simulink model "Comunicacao_Simulink_R2018b"  (R2018b)
settings: Solver=VariableStepAuto  StartTime=0.0  StopTime=10  RelTol=1e-3
libraries: dspsrcs4 x2, commsynccomp2 x1, simulink x1, dspmathops x1, commfilt2 x1, commutil2 x1
settings Model: Creator=rafae  LastModifiedBy=User

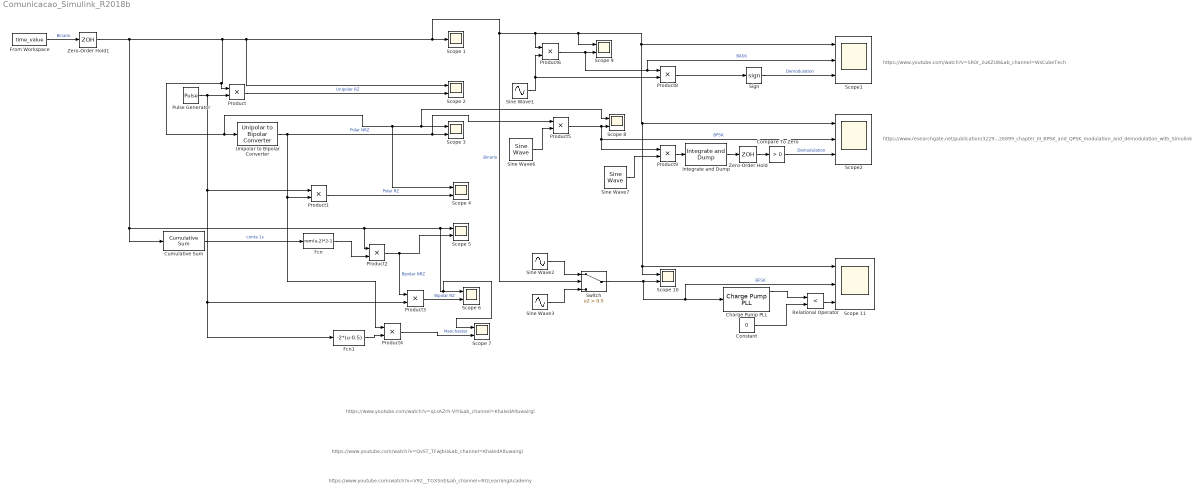
== system Comunicacao_Simulink_R2018b ==
  note: https://www.researchgate.net/publication/322926899_chapter_III_BPSK_and_QPSK_modulation_and_demodulation_with_Simulink
  note: https://www.youtube.com/watch?v=SR0r_2uKZU8&ab_channel=WsCubeTech
  note: https://www.youtube.com/watch?v=qLsAZrh-VIY&ab_channel=KhaledAltuwairgi
  note: https://www.youtube.com/watch?v=V92__TGXSnE&ab_channel=RGLearningAcademy
  note: https://www.youtube.com/watch?v=QvST_TFwJbU&ab_channel=KhaledAltuwairgi
  Charge Pump PLL : commsynccomp2/Charge Pump PLL  Fn=[2*pi*1]  Fd=[1 2*pi*1]  Kvco=4  Fc=10  Ph=0  Ac=1
      settings: SourceProductName=Communications Toolbox  SourceProductBaseCode=CM
  Compare To Zero : simulink/Logic and Bit Operations/Compare To Zero  relop=>  OutDataTypeStr=boolean
  Constant : Constant  Value=0
  Cumulative Sum : dspmathops/Cumulative Sum  dim=Channels (running sum)  InputProcessing=Columns as channels (frame based)  reset_popup=None  roundingMode=Floor  overflowMode=off  outputDataTypeStr=Inherit: Same as accumulator  outputMin=[]  outputMax=[]  outputLastDataTypeStr=Inherit: Same as accumulator
      settings: SourceProductName=DSP System Toolbox
  Fcn : Fcn  Expr=rem(u,2)*2-1
  Fcn1 : Fcn  Expr=-2*(u-0.5)
  From Workspace : FromWorkspace  VariableName=time_value  SampleTime=0
  Integrate and Dump : commfilt2/Integrate and Dump  obssamples=100  offsetsamples=0  nodump=on  roundingMode=Floor  overflowMode=off  outputDataTypeStr=Inherit: Same as accumulator  outputLastDataTypeStr=Inherit: Same as accumulator
      settings: SourceProductName=Communications Toolbox
  Product{,1..6,8..9} (9 alike) : Product
  Pulse Generator : DiscretePulseGenerator  PulseType=Time based  Period=1  PulseWidth=50
  Relational Operator : RelationalOperator  Operator=<  OutDataTypeStr=boolean  RndMeth=Simplest
  Scope 1 : Scope
  Scope {2..10} (9 alike) : Scope  NumInputPorts=2
  Scope 11 : Scope  NumInputPorts=3
  Scope1 : Scope  NumInputPorts=3
  Scope2 : Scope  NumInputPorts=3
  Sign : Signum
  Sine Wave1 : Sin  Frequency=2*pi*2  SampleTime=0
  Sine Wave2 : Sin  Frequency=2*pi*4  SampleTime=0
  Sine Wave3 : Sin  Frequency=2*pi*12  SampleTime=0
  Sine Wave6 : dspsrcs4/Sine Wave  Amplitude=1  Frequency=5  Phase=0  SampleMode=Discrete  OutComplex=Real  CompMethod=Trigonometric fcn  TableSize=Speed  SampleTime=1/1000  SamplesPerFrame=1  ResetState=Restart at time zero  OutputFrames=off  dataType=double  wordLen=16  udDataType=sfix(16)  fracBitsMode=Best precision  numFracBits=15  OutDataTypeStr=double  LastOutDataTypeStr=double
  Sine Wave7 : dspsrcs4/Sine Wave  Amplitude=1  Frequency=5  Phase=0  SampleMode=Discrete  OutComplex=Real  CompMethod=Trigonometric fcn  TableSize=Speed  SampleTime=1/1000  SamplesPerFrame=1  ResetState=Restart at time zero  OutputFrames=off  dataType=double  wordLen=16  udDataType=sfix(16)  fracBitsMode=Best precision  numFracBits=15  OutDataTypeStr=double  LastOutDataTypeStr=double
  Switch : Switch  Criteria=u2 > Threshold  Threshold=0.5
  Unipolar to Bipolar Converter : commutil2/Unipolar to Bipolar Converter  M=2  polarity=Positive  dataType=Inherit via internal rule
      settings: SourceProductName=Communications Toolbox
  Zero-Order Hold : ZeroOrderHold  SampleTime=-1
  Zero-Order Hold1 : ZeroOrderHold  SampleTime=-1
  wires:
  Zero-Order Hold1/1 -> Cumulative Sum/1, Product2/1, Scope 7/1, Scope 6/1, Scope 5/1, Scope 2/1, Switch/2, Scope2/1, Scope 10/1, Scope 11/1, Scope1/1, Scope 9/1, Product6/1, Scope 1/1, Scope 4/1, Scope 8/1, Scope 3/1, Unipolar to Bipolar Converter/1, Product/1  "Binario"
  Product/1 -> Scope 2/2  "Unipolar RZ"
  Unipolar to Bipolar Converter/1 -> Product4/1, Product1/2, Product5/1, Scope 3/2  "Polar NRZ"
  Product1/1 -> Scope 4/2  "Polar RZ"
  Cumulative Sum/1 -> Fcn/1  "conta 1s"
  Fcn/1 -> Product2/2
  Product2/1 -> Scope 5/2, Product3/1  "Bipolar NRZ"
  Pulse Generator/1 -> Fcn1/1, Product3/2, Product1/1, Product/2
  Product3/1 -> Scope 6/2  "Bipolar RZ"
  Fcn1/1 -> Product4/2
  Product4/1 -> Scope 7/2  "Manchester"
  Sine Wave1/1 -> Product6/2, Product8/2
  Product5/1 -> Product9/1, Scope2/2, Scope 8/2  "BPSK"
  Product6/1 -> Product8/1, Scope1/2, Scope 9/2  "BASK"
  Switch/1 -> Scope 10/2, Scope 11/2, Charge Pump PLL/1  "BFSK"
  Sine Wave2/1 -> Switch/1
  Sine Wave3/1 -> Switch/3
  Constant/1 -> Relational Operator/2
  Charge Pump PLL/1 -> Relational Operator/1
  Relational Operator/1 -> Scope 11/3
  Product8/1 -> Sign/1
  Sign/1 -> Scope1/3  "Demodulation"
  Product9/1 -> Integrate and Dump/1
  Integrate and Dump/1 -> Zero-Order Hold/1
  Zero-Order Hold/1 -> Compare To Zero/1
  Compare To Zero/1 -> Scope2/3  "Demodulation"
  Sine Wave7/1 -> Product9/2
  Sine Wave6/1 -> Product5/2
  From Workspace/1 -> Zero-Order Hold1/1  "Binario"
